simulink model "sampling"  (R2020a)
settings: Solver=VariableStepAuto  StartTime=0.0  StopTime=1  RelTol=1e-3
settings Model: Creator=Riyansh  LastModifiedBy=Riyansh

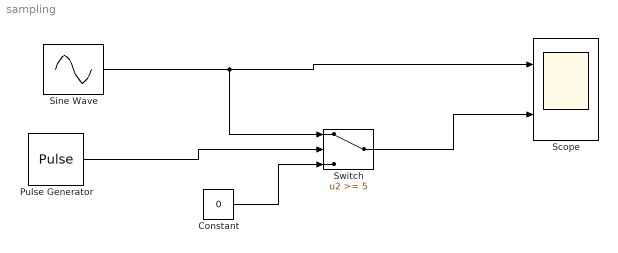
== system sampling ==
  Constant : Constant  Value=0
  Pulse Generator : DiscretePulseGenerator  PulseType=Time based  Amplitude=10  Period=0.01  PulseWidth=50
  Scope : Scope  NumInputPorts=2
  Sine Wave : Sin  Frequency=2*pi*5  SampleTime=1e-6
  Switch : Switch  Threshold=5
  wires:
  Sine Wave/1 -> Switch/1, Scope/1
  Pulse Generator/1 -> Switch/2
  Constant/1 -> Switch/3
  Switch/1 -> Scope/2
